simulink model "teoretsko_poredjenje_regulatora"  (R2015a)
settings: Solver=ode45  StartTime=0.0  StopTime=10.0  RelTol=1e-3
settings Model: Creator=Korisnik  LastModifiedBy=Korisnik

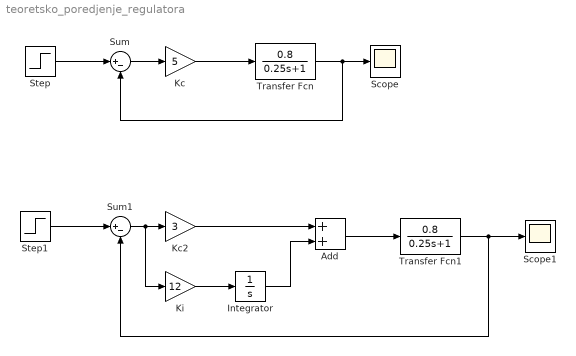
== system teoretsko_poredjenje_regulatora ==
  Add : Sum
  Integrator : Integrator
  Kc : Gain  Gain=5
  Kc2 : Gain  Gain=3
  Ki : Gain  Gain=12
  Scope : Scope
  Scope1 : Scope
  Step : Step  SampleTime=0
  Step1 : Step  SampleTime=0
  Sum : Sum  Inputs=|+-
  Sum1 : Sum  Inputs=|+-
  Transfer Fcn : TransferFcn  Numerator=[0.8]  Denominator=[0.25 1]
  Transfer Fcn1 : TransferFcn  Numerator=[0.8]  Denominator=[0.25 1]
  wires:
  Step/1 -> Sum/1
  Sum/1 -> Kc/1
  Kc/1 -> Transfer Fcn/1
  Transfer Fcn/1 -> Scope/1, Sum/2
  Step1/1 -> Sum1/1
  Sum1/1 -> Ki/1, Kc2/1
  Add/1 -> Transfer Fcn1/1
  Kc2/1 -> Add/1
  Transfer Fcn1/1 -> Sum1/2, Scope1/1
  Ki/1 -> Integrator/1
  Integrator/1 -> Add/2
